simulink model "ANSFT_Euler"  (R2023a)
settings: Solver=ode1  StartTime=0.0  StopTime=60  FixedStep=0.01  RelTol=1e-3
undefined symbols (not defined in the file or in its folder): HDBK, Light, MIL, sigbuilder_block
libraries: simulink x4, matrix_library x3, aerolibutil x3, robotcorelib x2, aerolibanim x1, simulink_extras x1, sharedtransform x1, aerolibwind2 x1, sim3dlib x1, uavsim3dlib x1
(part 2 of 2)

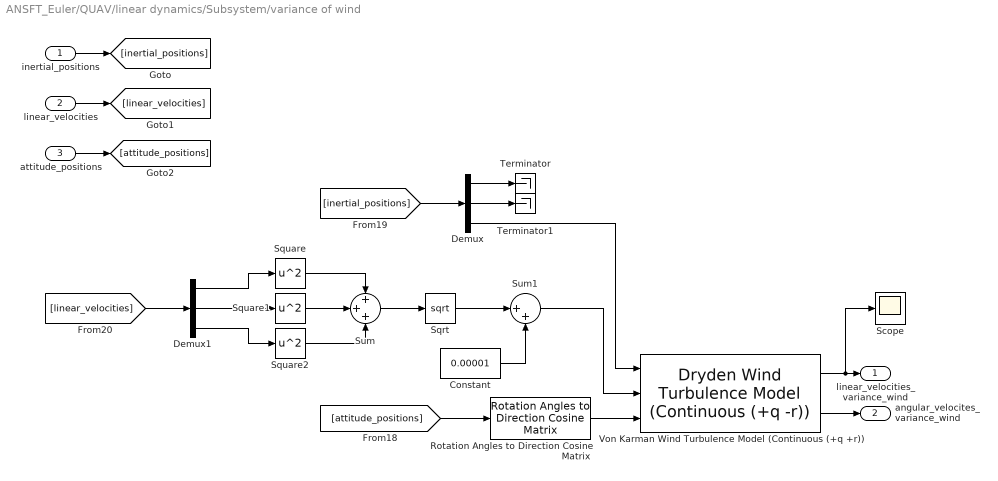
== system ANSFT_Euler/QUAV/linear dynamics/Subsystem/variance of wind ==
  inertial_positions : Inport
  linear_velocities : Inport  Port=2
  attitude_positions : Inport  Port=3
  Constant : Constant  Value=0.00001
  Demux : Demux  Outputs=3
  Demux1 : Demux  Outputs=3
  Rotation Angles to Direction Cosine Matrix : sharedtransform/Rotation Angles to Direction Cosine Matrix  rotationOrder=XYZ  aMode=aMode
  Scope : Scope
  Sqrt : Sqrt
  Square : Math  Operator=square
  Square1 : Math  Operator=square
  Square2 : Math  Operator=square
  Sum : Sum  Inputs=+++
  Sum1 : Sum  Inputs=|++
  Terminator : Terminator
  Terminator1 : Terminator
  Von Karman Wind Turbulence Model (Continuous (+q +r)) : aerolibwind2/Dryden Wind Turbulence Model  (Continuous (+q -r))  units=Metric (MKS)  spec=MIL-HDBK-1797  model=Continuous Von Karman (+q +r)  W20=15  Wdeg=0  TurbProb=10^-2 - Light  L_high=762  Wingspan=0.32  ts=0.1  Seed=[23341 23342 23343 23344]  T_on=on
      settings: LibrarySourceBlock=|
      | aerolibwind2/Von Karman Wind Turbulence Model
      | (Continuous (+q +r))
  linear_velocities_variance_wind : Outport
  angular_velocites_variance_wind : Outport  Port=2
  wires:
  Square1/1 -> Sum/2
  Demux1/1 -> Square/1
  Von Karman Wind Turbulence Model (Continuous (+q +r))/1 -> Scope/1, linear_velocities_variance_wind/1
  Demux/3 -> Von Karman Wind Turbulence Model (Continuous (+q +r))/1
  Sum/1 -> Sqrt/1
  [linear_velocities] -> Demux1/1
  Von Karman Wind Turbulence Model (Continuous (+q +r))/2 -> angular_velocites_variance_wind/1
  Square/1 -> Sum/1
  [attitude_positions] -> Rotation Angles to Direction Cosine Matrix/1
  Demux1/2 -> Square1/1
  Demux1/3 -> Square2/1
  Demux/2 -> Terminator1/1
  Square2/1 -> Sum/3
  Demux/1 -> Terminator/1
  Rotation Angles to Direction Cosine Matrix/1 -> Von Karman Wind Turbulence Model (Continuous (+q +r))/3
  [inertial_positions] -> Demux/1
  inertial_positions/1 -> [inertial_positions]
  linear_velocities/1 -> [linear_velocities]
  attitude_positions/1 -> [attitude_positions]
  Sqrt/1 -> Sum1/1
  Sum1/1 -> Von Karman Wind Turbulence Model (Continuous (+q +r))/2
  Constant/1 -> Sum1/2

== matlab function ANSFT_Euler/QUAV/linear dynamics/MATLAB Function2 ==
  data: attitude_positions input; y output
function y = rotationMatrix(attitude_positions)

roll = attitude_positions(1,1);
pitch = attitude_positions(2,1);
yaw = attitude_positions(3,1);

y = [
      cos(pitch)*cos(yaw) -cos(roll)*sin(yaw) + sin(roll)*sin(pitch)*cos(yaw)  sin(roll)*sin(yaw) + cos(roll)*sin(pitch)*cos(yaw);
      cos(pitch)*sin(yaw)  cos(roll)*cos(yaw) + sin(roll)*sin(pitch)*sin(yaw) -sin(roll)*cos(yaw) + cos(roll)*sin(pitch)*sin(yaw);
     -sin(pitch)           sin(roll)*cos(pitch)                                cos(roll)*cos(pitch)
    ];

== matlab function ANSFT_Euler/SVASMC/MATLAB Function2 ==
  data: pitch_parameter input; final_pitch_parameter output
function final_pitch_parameter = pitch_saturation(pitch_parameter)

if pitch_parameter > 1
    final_pitch_parameter = 1;
elseif pitch_parameter < -1
    final_pitch_parameter = -1;
else
    final_pitch_parameter = pitch_parameter;
end

% value_to_saturate = 0.3;
% 
% if pitch_parameter > value_to_saturate
%     final_pitch_parameter = value_to_saturate;
% elseif pitch_parameter < -value_to_saturate
%     final_pitch_parameter = -value_to_saturate;
% else
%     final_pitch_parameter = pitch_parameter;
% end

== matlab function ANSFT_Euler/QUAV/Subsystem/MATLAB Function ==
  data: attitude_positions input; inertial_angular_velocities output; body_angular_velocities input
function inertial_angular_velocities = body2inertial_angular(attitude_positions, body_angular_velocities)

roll = attitude_positions(1);
pitch = attitude_positions(2);

R2 = [1   sin(roll)*tan(pitch)    cos(roll)*tan(pitch);
      0   cos(roll)               -sin(roll);
      0   sin(roll)/cos(pitch)    cos(roll)/cos(pitch)];


inertial_angular_velocities = R2 * body_angular_velocities;

== matlab function ANSFT_Euler/SVASMC/MATLAB Function3 ==
  data: thrust input; final_thrust output
function final_thrust = thrust_saturation(thrust)

if thrust < -30
    final_thrust = -30;
elseif thrust > 0
    final_thrust = -1;
else 
    final_thrust = thrust;
end

== matlab function ANSFT_Euler/SVASMC/MATLAB Function4 ==
  data: roll_parameter input; final_roll_parameter output
function final_roll_parameter = roll_saturation(roll_parameter)

if roll_parameter > 1
    final_roll_parameter = 1;
elseif roll_parameter < -1
    final_roll_parameter = -1;
else
    final_roll_parameter = roll_parameter;
end

% The following is a more strict saturation, limiting the angles much more.
% value_to_saturate = 0.3;
% 
% if roll_parameter > value_to_saturate
%     final_roll_parameter = value_to_saturate;
% elseif roll_parameter < -value_to_saturate
%     final_roll_parameter = -value_to_saturate;
% else
%     final_roll_parameter = roll_parameter;
% end

== matlab function ANSFT_Euler/SVASMC/MATLAB Function5 ==
  data: thrust input; final_thrust output
function final_thrust = thrust_saturation(thrust)

if thrust < -30
    final_thrust = -30;
elseif thrust > 0
    final_thrust = -1;
else 
    final_thrust = thrust;
end
